simulink model "one_meter"  (R2023a)
settings: Solver=FixedStepDiscrete  StartTime=0.0  StopTime=10.0  FixedStep=0.01  RelTol=1e-3
libraries: arduinolib x3, mobileRoboticsTrainingLib x1
settings Model: SimulationMode=external  ExtModeTrigDuration=2  Creator=Jack Youens  LastModifiedBy=ankus
settings OptimizationCC: EnhancedBackFolding=on  PassReuseOutputArgsAs=Individual arguments  ZeroExternalMemoryAtStartup=off  ZeroInternalMemoryAtStartup=off  MaxStackSize=64  OptimizeBlockOrder=speed  DifferentSizesBufferReuse=on  OptimizationCustomize=off  EfficientTunableParamExpr=on
settings DebuggingCC: ParameterTunabilityLossMsg=error
settings HardwareCC: ProdBitPerPointer=32  ProdBitPerSizeT=32  ProdBitPerPtrDiffT=32  ProdLargestAtomicInteger=Long  ProdLargestAtomicFloat=Double  ProdWordSize=32  ProdHWDeviceType=ARM Compatible->ARM Cortex
settings SFSimCC: MATLABDynamicMemAlloc=off
settings RTWCC: Description=Embedded Coder  SystemTargetFile=ert.tlc  HardwareBoard=Arduino Nano 33 IoT  TemplateMakefile=ert_default_tmf  Toolchain=Arduino ARM  BuildConfiguration=Faster Runs
settings CodeAppCC: ForceParamTrailComments=on  IgnoreCustomStorageClasses=off  OperatorAnnotations=on  SimulinkDataObjDesc=on  SFDataObjDesc=on  InsertBlockDesc=on
settings ERTTargetCC: SupportContinuousTime=on  SupportVariableSizeSignals=on  ExtModeTransport=3  ExtModeStaticAlloc=on  ExtModeAutomaticAllocSize=off  ExtModeStaticAllocSize=8192  ExtModeMexFile=ext_xcp  ExtModeIntrfLevel=Level2 - Open

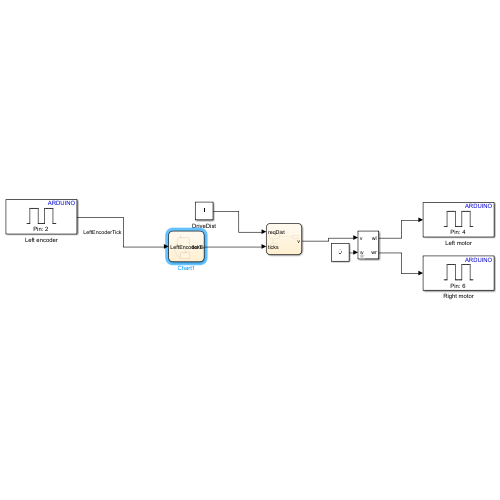
[thumbnail: Simulink's stored preview of the top-level diagram]
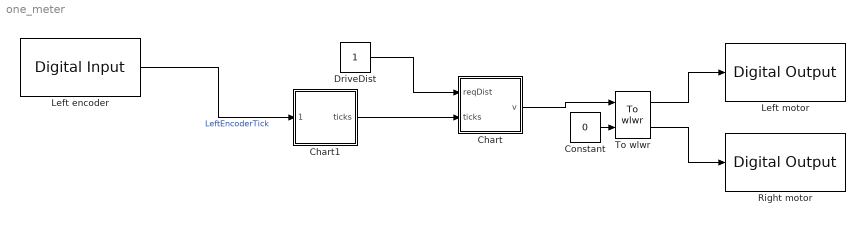
== system one_meter ==
  Chart : Stateflow chart  TreatAsAtomicUnit=on
  Chart1 : Stateflow chart  TreatAsAtomicUnit=on
  Constant : Constant  Value=0
  DriveDist : Constant
  Left encoder : arduinolib/Digital Input  pinNumber=2  mode=Default  Direction=input  SampleTime=0.1  blockPlatform=arduino
  Left motor : arduinolib/Digital Output  pinNumber=4  Direction=output  blockPlatform=arduino
  Right motor : arduinolib/Digital Output  pinNumber=6  Direction=output  blockPlatform=arduino
  To wlwr : mobileRoboticsTrainingLib/To wlwr  axleLength=0.1  wheelR=0.05
      link override change parameters: Gain=[1 -axleLength/2; 1 axleLength/2]
  wires:
  DriveDist/1 -> Chart/1(reqDist)
  Constant/1 -> To wlwr/2
  Chart/1(v) -> To wlwr/1
  Left encoder/1 -> Chart1/1(LeftEncoderTicks)  "LeftEncoderTick"
  Chart1/1(ticks) -> Chart/2(ticks)
  To wlwr/1 -> Left motor/1
  To wlwr/2 -> Right motor/1

== stateflow chart one_meter/Chart1 ==
  state Default
    entry:
    LeftEncoderTicks;
    ticks;
  state Accumulate
    entry:
    ticks = ticks + 1;
  (default) -> Default
  Accumulate -> Default
  Default -> Accumulate : [LeftEncoderTicks == 1]
  data: ticks output =0; LeftEncoderTicks input

== stateflow chart one_meter/Chart ==
  state Default
    entry:
    ticks;
    dist1Tick=(pi*0.031)/10
    reqTicks=reqDist/dist1Tick;
  state Stop
    entry:
    v=0;
  state Move
    entry:
    v=0.5;
  (default) -> Default
  Default -> Stop [order 2] : [ticks==reqTicks | ticks>reqTicks]
  Move -> Default
  Default -> Move [order 1] : [ticks<reqTicks]
  data: reqDist input; ticks input; v output; dist1Tick local; reqTicks local
